simulink library "sm_tractor_row_crop_lib"  (R2024b)
settings: Solver=VariableStepAuto  StartTime=0.0  StopTime=10.0  RelTol=1e-3
undefined symbols (not defined in the file): fluids, HMPST
libraries: fl_lib x88, nesl_utility x31, cvt_components_lib x25, sdl_lib x22, SimscapeFluids_lib x11, simulink_extras x5, $bdroot x4, ee_lib x2, batteryecm_lib x1, simulink x1, engine_mgmt_lib x1, slpidlib x1
(part 4 of 4)

== system sm_tractor_row_crop_lib/CVT Power Split Hydromechanical/Hydrostatic/Motor Leakage ==
  Case Drain : fl_lib/Isothermal Liquid/Elements/Reservoir (IL)  reservoir_type=foundation.enum.constant_controlled.constant  pressure_spec=foundation.enum.pressure_spec.atmospheric  reservoir_pressure=0.101325 MPa
  Leakage A : fl_lib/Isothermal Liquid/Elements/Laminar Leakage (IL)  cross_section_geometry=foundation.enum.cross_section_geometry.custom  diameter=1e-3 m  inner_diameter=5e-4 m  outer_diameter=1e-3 m  width=1e-3 m  height=0.1 m  major_axis=1e-3 m  minor_axis=5e-4 m  side_length=1e-3 m  length=5 m  resistance=1e7 s*MPa/m^3
      settings: InternalSimscapePortConfiguration="{\"Bottom\":[],\"Left\":[{\"id\":\"A\",\"label\":\"A\",\"type\":\"foundation.isothermal_liquid.isothermal_liquid\"}],\"Right\":[{\"id\":\"B\",\"label\":\"B\",\"type\":\"foundation.isothermal_liquid.isothermal_liquid\"}],\"Top\":[]}"
  Leakage B : fl_lib/Isothermal Liquid/Elements/Laminar Leakage (IL)  cross_section_geometry=foundation.enum.cross_section_geometry.custom  diameter=1e-3 m  inner_diameter=5e-4 m  outer_diameter=1e-3 m  width=1e-3 m  height=0.1 m  major_axis=1e-3 m  minor_axis=5e-4 m  side_length=1e-3 m  length=5 m  resistance=1e7 s*MPa/m^3
      settings: InternalSimscapePortConfiguration="{\"Bottom\":[],\"Left\":[{\"id\":\"A\",\"label\":\"A\",\"type\":\"foundation.isothermal_liquid.isothermal_liquid\"}],\"Right\":[{\"id\":\"B\",\"label\":\"B\",\"type\":\"foundation.isothermal_liquid.isothermal_liquid\"}],\"Top\":[]}"
  A : PMIOPort  Side=Left
  B : PMIOPort  Port=2  Side=Left
  connections:
  Leakage A/LConn1 -- A/RConn1
  Leakage B/RConn1 -- Case Drain/LConn1 -- Leakage A/RConn1
  Leakage B/LConn1 -- B/RConn1

== system sm_tractor_row_crop_lib/CVT Power Split Hydromechanical/Hydrostatic/Pump Leakage ==
  Case Drain : fl_lib/Isothermal Liquid/Elements/Reservoir (IL)  reservoir_type=foundation.enum.constant_controlled.constant  pressure_spec=foundation.enum.pressure_spec.atmospheric  reservoir_pressure=0.101325 MPa
  Leakage A : fl_lib/Isothermal Liquid/Elements/Laminar Leakage (IL)  cross_section_geometry=foundation.enum.cross_section_geometry.custom  diameter=1e-3 m  inner_diameter=5e-4 m  outer_diameter=1e-3 m  width=1e-3 m  height=0.1 m  major_axis=1e-3 m  minor_axis=5e-4 m  side_length=1e-3 m  length=5 m  resistance=1e7 s*MPa/m^3
      settings: InternalSimscapePortConfiguration="{\"Bottom\":[],\"Left\":[{\"id\":\"A\",\"label\":\"A\",\"type\":\"foundation.isothermal_liquid.isothermal_liquid\"}],\"Right\":[{\"id\":\"B\",\"label\":\"B\",\"type\":\"foundation.isothermal_liquid.isothermal_liquid\"}],\"Top\":[]}"
  Leakage B : fl_lib/Isothermal Liquid/Elements/Laminar Leakage (IL)  cross_section_geometry=foundation.enum.cross_section_geometry.custom  diameter=1e-3 m  inner_diameter=5e-4 m  outer_diameter=1e-3 m  width=1e-3 m  height=0.1 m  major_axis=1e-3 m  minor_axis=5e-4 m  side_length=1e-3 m  length=5 m  resistance=1e7 s*MPa/m^3
      settings: InternalSimscapePortConfiguration="{\"Bottom\":[],\"Left\":[{\"id\":\"A\",\"label\":\"A\",\"type\":\"foundation.isothermal_liquid.isothermal_liquid\"}],\"Right\":[{\"id\":\"B\",\"label\":\"B\",\"type\":\"foundation.isothermal_liquid.isothermal_liquid\"}],\"Top\":[]}"
  B : PMIOPort  Side=Left
  A : PMIOPort  Port=2  Side=Left
  connections:
  Leakage A/LConn1 -- A/RConn1
  Leakage B/RConn1 -- Leakage A/RConn1 -- Case Drain/LConn1
  Leakage B/LConn1 -- B/RConn1

== system sm_tractor_row_crop_lib/Controller/CVT Ratio Ctrl/Range Calculation ==
  Ratio (-) : Inport
  Check Range 0 or higher : Switch  Threshold=XY_I(1,2)  SaturateOnIntegerOverflow=off  InputSameDT=off
  Check Range 2 or higher : Switch  Threshold=XY_I(2,2)  SaturateOnIntegerOverflow=off  InputSameDT=off
  Check Range 3 or higher : Switch  Threshold=XY_I(3,2)  SaturateOnIntegerOverflow=off  InputSameDT=off
  Check Range 4 : Switch  Threshold=XY_I(4,2)  SaturateOnIntegerOverflow=off  InputSameDT=off
  Constant1 : Constant  Value=2  SampleTime=HMPST.Simu.TimeStep
  Constant2 : Constant  SampleTime=HMPST.Simu.TimeStep
  Constant3 : Constant  Value=-1  SampleTime=HMPST.Simu.TimeStep
  Constant4 : Constant  Value=3  SampleTime=HMPST.Simu.TimeStep
  Constant5 : Constant  Value=4  SampleTime=HMPST.Simu.TimeStep
  Range (-) : Outport
  wires:
  Check Range 2 or higher/1 -> Check Range 0 or higher/1
  Constant2/1 -> Check Range 2 or higher/3
  Constant3/1 -> Check Range 0 or higher/3
  Check Range 0 or higher/1 -> Range (-)/1  "Range"
  Check Range 3 or higher/1 -> Check Range 2 or higher/1
  Constant1/1 -> Check Range 3 or higher/3
  Check Range 4/1 -> Check Range 3 or higher/1
  Constant4/1 -> Check Range 4/3
  Constant5/1 -> Check Range 4/1
  Ratio (-)/1 -> Check Range 2 or higher/2, Check Range 3 or higher/2, Check Range 4/2, Check Range 0 or higher/2

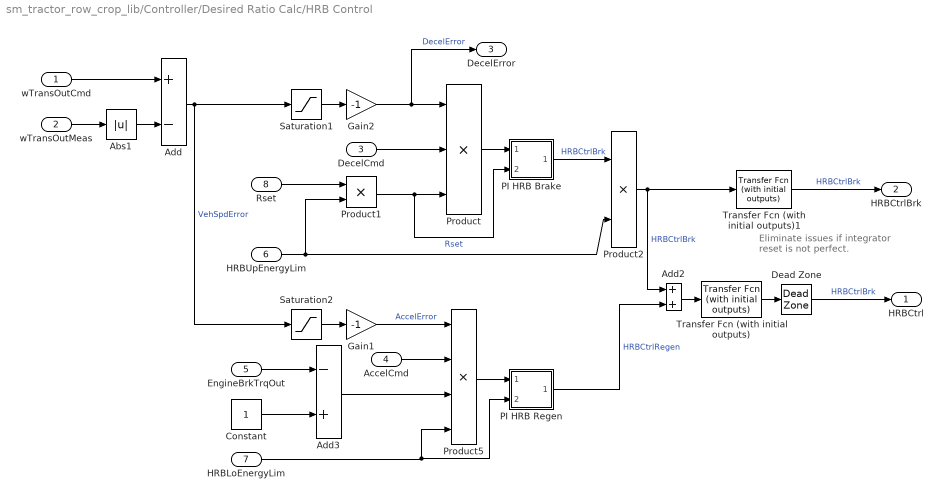
== system sm_tractor_row_crop_lib/Controller/Desired Ratio Calc/HRB Control ==
  note: Eliminate issues if integrator reset is not perfect.
  wTransOutCmd : Inport
  wTransOutMeas : Inport  Port=2
  DecelCmd : Inport  Port=3
  AccelCmd : Inport  Port=4
  EngineBrkTrqOut : Inport  Port=5
  HRBUpEnergyLim : Inport  Port=6
  HRBLoEnergyLim : Inport  Port=7
  Rset : Inport  Port=8
  Abs1 : Abs  ZeroCross=off  SaturateOnIntegerOverflow=off
  Add : Sum  Inputs=+-
  Add2 : Sum
  Add3 : Sum  Inputs=-+
  Constant : Constant
  Dead Zone : DeadZone  LowerValue=-3e-3  UpperValue=3e-3
  Gain1 : Gain  Gain=-1
  Gain2 : Gain  Gain=-1
  PI HRB Brake : Subsystem
  PI HRB Regen : Subsystem
  Product : Product  Inputs=3
  Product1 : Product
  Product2 : Product
  Product5 : Product  Inputs=4
  Saturation1 : Saturate  UpperLimit=0  LowerLimit=-inf  ZeroCross=off
  Saturation2 : Saturate  UpperLimit=inf  LowerLimit=0  ZeroCross=off
  Transfer Fcn (with initial outputs) : simulink_extras/Additional Linear/Transfer Fcn (with initial outputs)  N=[0.01]  D=[0.05 1]  Y0=0  U0=0
  Transfer Fcn (with initial outputs)1 : simulink_extras/Additional Linear/Transfer Fcn (with initial outputs)  N=[0.01]  D=[0.05 1]  Y0=0  U0=0
  HRBCtrl : Outport
  HRBCtrlBrk : Outport  Port=2
  DecelError : Outport  Port=3
  wires:
  Transfer Fcn (with initial outputs)/1 -> Dead Zone/1
  Product/1 -> PI HRB Brake/1(error)
  Product5/1 -> PI HRB Regen/1(error)
  Gain1/1 -> Product5/1  "AccelError"
  Transfer Fcn (with initial outputs)1/1 -> HRBCtrlBrk/1  "HRBCtrlBrk"
  Rset/1 -> Product1/1
  EngineBrkTrqOut/1 -> Add3/1
  wTransOutCmd/1 -> Add/1
  PI HRB Brake/1(ctrl) -> Product2/1  "HRBCtrlBrk"
  wTransOutMeas/1 -> Abs1/1
  Gain2/1 -> Product/1, DecelError/1  "DecelError"
  AccelCmd/1 -> Product5/2
  Saturation1/1 -> Gain2/1
  Saturation2/1 -> Gain1/1
  PI HRB Regen/1(ctrl) -> Add2/2  "HRBCtrlRegen"
  HRBUpEnergyLim/1 -> Product2/2, Product1/2
  Abs1/1 -> Add/2
  DecelCmd/1 -> Product/2
  Product2/1 -> Add2/1, Transfer Fcn (with initial outputs)1/1  "HRBCtrlBrk"
  Add/1 -> Saturation1/1, Saturation2/1  "VehSpdError"
  Dead Zone/1 -> HRBCtrl/1  "HRBCtrlBrk"
  Constant/1 -> Add3/2
  Product1/1 -> Product/3, PI HRB Brake/2(Rset)  "Rset"
  Add3/1 -> Product5/3
  HRBLoEnergyLim/1 -> Product5/4, PI HRB Regen/2(Rset)
  Add2/1 -> Transfer Fcn (with initial outputs)/1

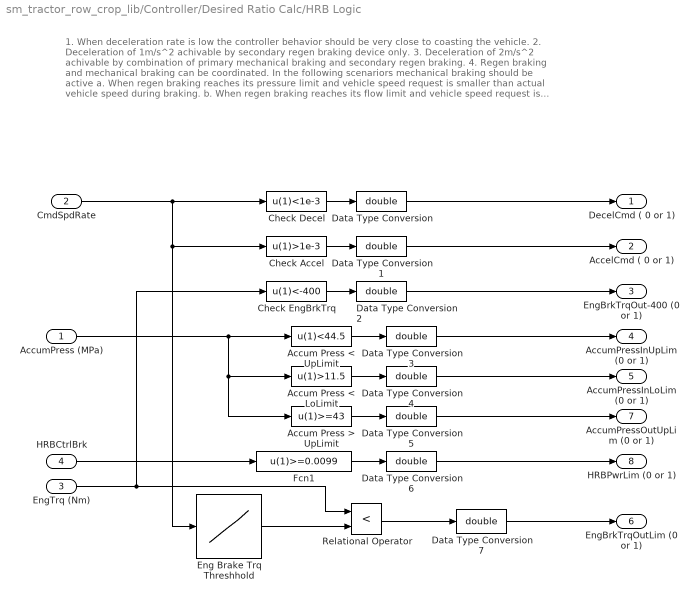
== system sm_tractor_row_crop_lib/Controller/Desired Ratio Calc/HRB Logic ==
  note: 1. When deceleration rate is low the controller behavior should be very close to coasting the vehicle.
      | 2. Deceleration of 1m/s^2 achivable by secondary regen braking device only.
      | 3. Deceleration of 2m/s^2 achivable by combination of primary mechanical braking and secondary regen braking.
      | 4. Regen braking and mechanical braking can be coordinated. In the following scenariors mechanical braking should be active
      | a. When regen braking reaches its pressure limit and vehicle speed request is smaller than actual vehicle speed during braking.
      | b. When regen braking reaches its flow limit and vehicle speed request is smaller than actual vehicle speed during braking.
      | 5. Energy in the accumulator will be released when accelerating and the accumulator pressure is above minimum working pressure.
      | Energy release rate should not cause engine over speeding.
      | 6. If engine over speed limit is reached disengage master clutch/shut down the engine.
  AccumPress (MPa) : Inport
  CmdSpdRate : Inport  Port=2
  EngTrq (Nm) : Inport  Port=3
  HRBCtrlBrk : Inport  Port=4
  Accum Press < LoLimit : Fcn  Expr=u(1)>11.5
  Accum Press < UpLimit : Fcn  Expr=u(1)<44.5
  Accum Press > UpLimit : Fcn  Expr=u(1)>=43
  Check Accel : Fcn  Expr=u(1)>1e-3
  Check Decel : Fcn  Expr=u(1)<1e-3
  Check EngBrkTrq : Fcn  Expr=u(1)<-400
  Data Type Conversion{,1..7} (8 alike) : DataTypeConversion  OutDataTypeStr=double  SaturateOnIntegerOverflow=off  RndMeth=Floor
  Eng Brake Trq Threshhold : Lookup_n-D  NumberOfTableDimensions=1  BreakpointsForDimension1=[-3 -2 -1 -0.5 0 1]  Table=[-450 -450 -225 -113 0 0]*0.6  InternalRulePriority=Speed  RndMeth=Simplest
  Fcn1 : Fcn  Expr=u(1)>=0.0099
  Relational Operator : RelationalOperator  Operator=<  OutDataTypeStr=boolean  ZeroCross=off  InputSameDT=off
  DecelCmd ( 0 or 1) : Outport
  AccelCmd ( 0 or 1) : Outport  Port=2
  EngBrkTrqOut-400 (0 or 1) : Outport  Port=3
  AccumPressInUpLim (0 or 1) : Outport  Port=4
  AccumPressInLoLim (0 or 1) : Outport  Port=5
  EngBrkTrqOutLim (0 or 1) : Outport  Port=6
  AccumPressOutUpLim (0 or 1) : Outport  Port=7
  HRBPwrLim (0 or 1) : Outport  Port=8
  wires:
  Check Decel/1 -> Data Type Conversion/1
  Data Type Conversion/1 -> DecelCmd ( 0 or 1)/1
  EngTrq (Nm)/1 -> Relational Operator/1, Check EngBrkTrq/1
  CmdSpdRate/1 -> Check Decel/1, Eng Brake Trq Threshhold/1, Check Accel/1
  Eng Brake Trq Threshhold/1 -> Relational Operator/2
  AccumPress (MPa)/1 -> Accum Press < LoLimit/1, Accum Press > UpLimit/1, Accum Press < UpLimit/1
  Accum Press < UpLimit/1 -> Data Type Conversion3/1
  Relational Operator/1 -> Data Type Conversion7/1
  Accum Press > UpLimit/1 -> Data Type Conversion5/1
  HRBCtrlBrk/1 -> Fcn1/1
  Fcn1/1 -> Data Type Conversion6/1
  Accum Press < LoLimit/1 -> Data Type Conversion4/1
  Check Accel/1 -> Data Type Conversion1/1
  Check EngBrkTrq/1 -> Data Type Conversion2/1
  Data Type Conversion1/1 -> AccelCmd ( 0 or 1)/1
  Data Type Conversion2/1 -> EngBrkTrqOut-400 (0 or 1)/1
  Data Type Conversion3/1 -> AccumPressInUpLim (0 or 1)/1
  Data Type Conversion4/1 -> AccumPressInLoLim (0 or 1)/1
  Data Type Conversion5/1 -> AccumPressOutUpLim (0 or 1)/1
  Data Type Conversion6/1 -> HRBPwrLim (0 or 1)/1
  Data Type Conversion7/1 -> EngBrkTrqOutLim (0 or 1)/1

== system sm_tractor_row_crop_lib/Controller/Desired Ratio Calc/MB Control ==
  Decel Error : Inport
  wTransOutCmd : Inport  Port=2
  Rset : Inport  Port=3
  AccumLimUp : Inport  Port=4
  HRBPowerLim : Inport  Port=5
  Add1 : Sum  Inputs=+++
  Compare To Constant : simulink/Logic and Bit Operations/Compare To Constant  relop=<=  const=0.02  OutDataTypeStr=boolean
  Data Type Conversion : DataTypeConversion  OutDataTypeStr=double  SaturateOnIntegerOverflow=off  RndMeth=Floor
  PI MB No HRB : Subsystem
  PI MB with MRB : Subsystem
  Product3 : Product  Inputs=3
  Product4 : Product
  Out1 : Outport
  wires:
  HRBPowerLim/1 -> Product4/2
  AccumLimUp/1 -> Product3/3
  wTransOutCmd/1 -> Compare To Constant/1
  PI MB with MRB/1(ctrl) -> Add1/3
  Add1/1 -> Out1/1
  Product4/1 -> PI MB with MRB/1(error)
  PI MB No HRB/1(ctrl) -> Add1/2
  Data Type Conversion/1 -> Add1/1
  Compare To Constant/1 -> Data Type Conversion/1
  Rset/1 -> PI MB with MRB/2(Rset), PI MB No HRB/2(Rset), Product3/2
  Product3/1 -> PI MB No HRB/1(error)
  Decel Error/1 -> Product4/1, Product3/1

== system sm_tractor_row_crop_lib/Controller/Desired Ratio Calc/VehSpdDir ==
  u : Inport
  Constant1 : Constant
  Constant2 : Constant  Value=-1
  Constant3 : Constant  Value=0
  Gain : Gain  Gain=-1
  Switch : Switch  Criteria=u2 > Threshold  Threshold=0.001  SaturateOnIntegerOverflow=off  InputSameDT=off
  Switch1 : Switch  Criteria=u2 > Threshold  Threshold=0.001  SaturateOnIntegerOverflow=off  InputSameDT=off
  u_dir : Outport
  wires:
  Gain/1 -> Switch1/2
  Switch/1 -> u_dir/1
  u/1 -> Switch/2, Gain/1
  Constant1/1 -> Switch/1
  Switch1/1 -> Switch/3
  Constant3/1 -> Switch1/3
  Constant2/1 -> Switch1/1

== system sm_tractor_row_crop_lib/Controller/Desired Ratio Calc/HRB Control/PI HRB Brake ==
  error : Inport
  Rset : Inport  Port=2
  Gain : Gain  Gain=0.02*0.2
  Gain3 : Gain  Gain=0.002+0.0005
  Integrator : Integrator  ExternalReset=falling
  Sum : Sum  Inputs=++|
  ctrl : Outport
  wires:
  Rset/1 -> Integrator/2
  Integrator/1 -> Sum/1
  error/1 -> Gain3/1, Gain/1
  Sum/1 -> ctrl/1
  Gain3/1 -> Integrator/1
  Gain/1 -> Sum/2

== system sm_tractor_row_crop_lib/Controller/Desired Ratio Calc/HRB Control/PI HRB Regen ==
  error : Inport
  Rset : Inport  Port=2
  Gain : Gain  Gain=0.01*0.2
  Gain3 : Gain  Gain=0.001
  Integrator : Integrator  ExternalReset=falling
  Sum : Sum  Inputs=++|
  ctrl : Outport
  wires:
  Gain/1 -> Sum/2
  Gain3/1 -> Integrator/1
  Sum/1 -> ctrl/1
  error/1 -> Gain/1, Gain3/1
  Integrator/1 -> Sum/1
  Rset/1 -> Integrator/2

== system sm_tractor_row_crop_lib/Controller/Desired Ratio Calc/MB Control/PI MB No HRB ==
  error : Inport
  Rset : Inport  Port=2
  Gain : Gain  Gain=0.01
  Gain3 : Gain  Gain=0.002
  Integrator : Integrator  ExternalReset=falling
  Sum : Sum  Inputs=++|
  ctrl : Outport
  wires:
  Rset/1 -> Integrator/2
  Integrator/1 -> Sum/1
  error/1 -> Gain3/1, Gain/1
  Sum/1 -> ctrl/1
  Gain3/1 -> Integrator/1
  Gain/1 -> Sum/2

== system sm_tractor_row_crop_lib/Controller/Desired Ratio Calc/MB Control/PI MB with MRB ==
  error : Inport
  Rset : Inport  Port=2
  Gain : Gain  Gain=0.005
  Gain3 : Gain  Gain=0.002
  Integrator : Integrator  ExternalReset=falling
  Sum : Sum  Inputs=++|
  ctrl : Outport
  wires:
  Gain/1 -> Sum/2
  Gain3/1 -> Integrator/1
  Sum/1 -> ctrl/1
  error/1 -> Gain/1, Gain3/1
  Integrator/1 -> Sum/1
  Rset/1 -> Integrator/2

== stateflow chart sm_tractor_row_crop_lib/Controller/CVT Ratio Ctrl/Clutch Truth Table ==
  state ClutchLogic
    during:
    [K1Actv,K2Actv,K3Actv,K4Actv,KbActv] = ClutchTable(Range);
    state Rest
      during:
      KvActv = 0;
      KrActv = 0;
    state Fwd
      during:
      KvActv = 1;
      KrActv = 0;
    state Rev
      during:
      KvActv = 0;
      KrActv = 1;
    (default) -> (junction 53)
    (junction 53) -> Fwd [order 3]
    (junction 53) -> Rev [order 2] : [CmdVehSpdDir==-1]
    (junction 53) -> Rest [order 1] : [CmdVehSpdDir==0]
    Fwd -> Rest : [CmdVehSpdDir~=1]
    Rev -> Rest : [CmdVehSpdDir~=-1]
    Rest -> Fwd [order 1] : [CmdVehSpdDir==1]
    Rest -> Rev [order 2] : [CmdVehSpdDir==-1]
  data: R function_input; K1 function_output; K2 function_output; K3 function_output; K4 function_output; Kb function_output; Range input; K1Actv output; K2Actv output; K3Actv output; K4Actv output; KbActv output; KvActv output; KrActv output; CmdVehSpdDir input
  function [K1,K2,K3,K4,Kb] = ClutchTable(R):
    | function [K1,K2,K3,K4,Kb] = ClutchTable(R)
    | 
    | aVarTruthTableCondition_1 = false;
    | aVarTruthTableCondition_2 = false;
    | aVarTruthTableCondition_3 = false;
    | aVarTruthTableCondition_4 = false;
    | 
    | 
    | % Range1
    | 
    | aVarTruthTableCondition_1 = logical(R == 1);
    | 
    | % Range2
    | 
    | aVarTruthTableCondition_2 = logical(R == 2);
    | 
    | % Range3
    | 
    | aVarTruthTableCondition_3 = logical(R == 3);
    | 
    | % Range4
    | 
    | aVarTruthTableCondition_4 = logical(R == 4);
    | 
    | if (aVarTruthTableCondition_1 && ~aVarTruthTableCondition_2 && ~aVarTruthTableCondition_3 && ~aVarTruthTableCondition_4)
    |     A1();
    | elseif (~aVarTruthTableCondition_1 && aVarTruthTableCondition_2 && ~aVarTruthTableCondition_3 && ~aVarTruthTableCondition_4)
    |     A2();
    | elseif (~aVarTruthTableCondition_1 && ~aVarTruthTableCondition_2 && aVarTruthTableCondition_3 && ~aVarTruthTableCondition_4)
    |     A3();
    | elseif (~aVarTruthTableCondition_1 && ~aVarTruthTableCondition_2 && ~aVarTruthTableCondition_3 && aVarTruthTableCondition_4)
    |     A4();
    | else % Default
    |     A5();
    | end
    | 
    | function A1()
    | 
    | % ClutchCtrlR1
    | 
    | K1 = 1; K2 = 0; K3 = 0; K4 = 0; Kb = 1;
    | 
    | function A2()
    | 
    | % ClutchCtrlR2
    | 
    | K1 = 0; K2 = 1; K3 = 0; K4 = 0; Kb = 1;
    | 
    | function A3()
    | 
    | % ClutchCtrlR3
    | 
    | K1 = 0; K2 = 1; K3 = 1; K4 = 0; Kb = 0;
    | 
    | function A4()
    | 
    | % ClutchCtrlR4
    | 
    | K1 = 0; K2 = 1; K3 = 0; K4 = 1; Kb = 0;
    | 
    | function A5()
    | 
    | % Default
    | 
    | K1 = 0; K2 = 0; K3 = 0; K4 = 0; Kb = 0;
